simulink model "tdk_sim"  (R2017a)
settings: Solver=ode4  StartTime=0.0  StopTime=10  FixedStep=0.01  MaxStep=0.05  RelTol=1e-3  EnableMultiTasking=on
values from neighbouring files (symbols this model uses):
  x0_tdk = [0.5 0.5 0 0.1 0 0 0 0 0 0]    [tdk_sim_ini.m]
settings Model: Creator=ut  LastModifiedBy=maam
settings DataIOCC: LimitDataPoints=on  SaveFormat=Array  SignalLoggingSaveFormat=ModelDataLogs
settings OptimizationCC: ExpressionDepthLimit=2147483647  InitFltsAndDblsToZero=on  LifeSpan=inf
settings DebuggingCC: SaveWithParameterizedLinksMsg=none  UnderspecifiedInitializationDetection=Classic  MergeDetectMultiDrivingBlocksExec=none  SignalResolutionControl=TryResolveAllWithWarning  SolverPrmCheckMsg=warning  MultiTaskDSMMsg=warning  MultiTaskCondExecSysMsg=none  FcnCallInpInsideContextMsg=warning  StateNameClashWarn=warning  SFUnexpectedBacktrackingDiag=warning  SFNoUnconditionalDefaultTransitionDiag=warning  SFExecutionAtInitializationDiag=none
settings HardwareCC: ProdBitPerPointer=32  ProdBitPerSizeT=32  ProdBitPerPtrDiffT=32  ProdLargestAtomicFloat=None  ProdIntDivRoundTo=Undefined  ProdEndianess=Unspecified  ProdWordSize=32  ProdHWDeviceType=32-bit Generic
settings ModelReferenceCC: PropagateSignalLabelsOutOfModel=off
settings GRTTargetCC: TargetFcnLib=ansi_tfl_tmw.mat  TargetLangStandard=C89/C90 (ANSI)  CombineOutputUpdateFcns=off  GRTInterface=on
settings ConfigComp: CovMetricSettings=dw  CovSaveCumulativeToWorkspaceVar=on  CovSaveSingleToWorkspaceVar=on  CovExternalEMLEnable=off

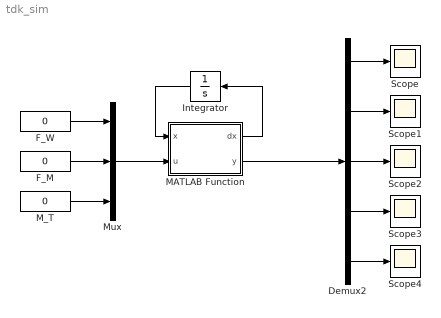
== system tdk_sim ==
  Demux2 : Demux  Outputs=5
  F_M : Constant  Value=0
  F_W : Constant  Value=0
  Integrator : Integrator  InitialCondition=x0_tdk
  MATLAB Function : MATLAB Function  TreatAsAtomicUnit=on
  M_T : Constant  Value=0
  Mux : Mux  Inputs=3
  Scope{,1..4} (5 alike) : Scope
  wires:
  MATLAB Function/2(y) -> Demux2/1
  Demux2/1 -> Scope/1
  Demux2/2 -> Scope1/1
  Demux2/3 -> Scope2/1
  Demux2/4 -> Scope3/1
  Demux2/5 -> Scope4/1
  MATLAB Function/1(dx) -> Integrator/1
  Integrator/1 -> MATLAB Function/1(x)
  F_W/1 -> Mux/1
  F_M/1 -> Mux/2
  M_T/1 -> Mux/3
  Mux/1 -> MATLAB Function/2(u)

== matlab function tdk_sim/MATLAB Function ==
  data: dx output; x input; y output; u input; par_tdk parameter
function [dx, y] = tdk_fcn(x, u, par_tdk)
%
% inputs:   u1(1)... F_W   Force of the cart [N]
%           u2(1)... F_M   Force of the rope winch [N]
%           u3(1)... M_T   Torque of the tower [Nm]
%
% states:   x(1)... l_W          Position of the cart [m]
%           x(2)... l_s          Rope length [m]
%           x(3)... phi_zi       Angle of the tower [rad]
%           x(4)... phi_xt       Angle of the load (x-axis) [rad]
%           x(5)... phi_yt       Angle of the load (y-axis) [rad]
%           x(6)... dot(l_W)     Velocity of the cart [m/s]
%           x(7)... dot(l_s)     Velocity of the rope [m/s]
%           x(8)... dot(phi_zi)  Angular velocity of the tower [rad/s]
%           x(9)... dot(phi_xt)  Angular velocity of the load (x-axis) [rad/s]
%           x(10)... dot(phi_yt) Angular velocity of the load (y-axis) [rad/s]
%
% outputs:  y(1)... l_W          Position of the cart [m]
%           y(2)... l_s          Rope length [m]
%           y(3)... phi_zi       Angle of the tower [rad]
%           y(4)... phi_xt       Angle of the load (x-axis) [rad]
%           y(5)... phi_yt       Angle of the load (y-axis) [rad]
%
% parameter: par_tdk(1)... m_M     Mass o the load m [kg]
%            par_tdk(2)... m_W     Mass of the cart
%            par_tdk(3)... m_TA    Mass of the tower-cantilever unit (TC-unit)
%            par_tdk(4)... k_M     Friction coefficient of the load
%            par_tdk(5)... k_TA    Friction coefficient of the load TC-unit
%            par_tdk(6)... k_W     Friction coefficient of the cart
%            par_tdk(7)... hTA     Height of the center of gravity of the TC-unit
%            par_tdk(8)... lTA     Distance of the center of gravity of the TC-unit in yi-direction
%            par_tdk(9)... J_Wzz   Inertia tensor of the cart
%            par_tdk(10)... J_TAzz Inertia tensor of the TC-unit
%            par_tdk(11)... g      Gravity acceleration
%    
    % Reading the model parameters               
    m_M = par_tdk(1); 
    m_W = par_tdk(2);  
    m_TA = par_tdk(3);  
    k_M = par_tdk(4); 
    k_TA = par_tdk(5); 
    k_W = par_tdk(6); 
    hTA = par_tdk(7); 
    lTA = par_tdk(8); 
    J_Wzz = par_tdk(9); 
    J_TAzz = par_tdk(10); 
    g = par_tdk(11);          

    % Shortcut for the inputs
    F_W = u(1);
    F_M = u(2);
    M_T = u(3);


    % Substitutions
    x_1 = x(1);
    x_2 = x(2);
    x_3 = x(3);
    x_4 = x(4);
    x_5 = x(5);
    x_6 = x(6);
    x_7 = x(7);
    x_8 = x(8);
    x_9 = x(9);
    x_10 = x(10);  

    % Calculation of the states time derivative
    dx = zeros(10, 1);
    dx(1) = x_6;
    dx(2) = x_7;
    dx(3) = x_8;
    dx(4) = x_9;
    dx(5) = x_10;
    dx(6) = (x_1*x_2*x_8^2*m_W-x_2*x_6*k_W-cos(x_4)*x_9*k_M+x_2*F_W)/(x_2*m_W);
    dx(7) = (x_1*x_2*cos(x_4)*sin(x_5)*m_M*m_W*M_T+(x_1^2*(x_2^2*(x_9^2+x_8*(2*sin(x_5)*x_9-2*x_10*cos(x_4)*sin(x_4)*cos(x_5))+(1-cos(x_4)^2*cos(x_5)^2)*x_8^2+x_10^2*cos(x_4)^2)+g*x_2*cos(x_4)*cos(x_5))*m_M-x_1^2*x_2*F_M)*m_W^2+((((x_2^2*(x_9^2+x_8*(2*sin(x_5)*x_9-2*x_10*cos(x_4)*sin(x_4)*cos(x_5))+(1-cos(x_4)^2*cos(x_5)^2)*x_8^2+x_10^2*cos(x_4)^2)+g*x_2*cos(x_4)*cos(x_5))*lTA^2-2*x_2*cos(x_4)*sin(x_5)*x_6*x_8*lTA^2)*m_M-x_2*F_M*lTA^2)*m_TA+(x_6*((-2*J_Wzz-2*J_TAzz)*x_2*cos(x_4)*sin(x_5)*x_8-x_1^2*x_2*sin(x_4)*k_W)+x_1*x_2*(cos(x_4)*sin(x_5)*x_8*k_TA+(cos(x_4)*cos(x_5)^2*x_9-cos(x_4)*x_9+x_10*sin(x_4)*cos(x_5)*sin(x_5))*k_M)+x_1^2*((-cos(x_4)*sin(x_4)*cos(x_5)^2*x_9-x_10*cos(x_5)*sin(x_5))*k_M+x_2*sin(x_4)*F_W)+x_2^2*((J_Wzz+J_TAzz)*x_9^2+x_8*((2*J_Wzz+2*J_TAzz)*sin(x_5)*x_9+(-2*J_Wzz-2*J_TAzz)*x_10*cos(x_4)*sin(x_4)*cos(x_5))+((-J_Wzz-J_TAzz)*cos(x_4)^2*cos(x_5)^2+J_Wzz+J_TAzz)*x_8^2+(J_Wzz+J_TAzz)*x_10^2*cos(x_4)^2)+(g*J_Wzz+g*J_TAzz)*x_2*cos(x_4)*cos(x_5))*m_M+(-J_Wzz-J_TAzz)*x_2*F_M)*m_W+((x_2*sin(x_4)*F_W-cos(x_4)*sin(x_4)*x_9*k_M)*lTA^2-x_2*sin(x_4)*x_6*k_W*lTA^2)*m_M*m_TA+((-J_Wzz-J_TAzz)*x_2*sin(x_4)*x_6*k_W+(-J_Wzz-J_TAzz)*cos(x_4)*sin(x_4)*x_9*k_M+(J_Wzz+J_TAzz)*x_2*sin(x_4)*F_W)*m_M)/(x_1^2*x_2*m_M*m_W^2+(x_2*lTA^2*m_M*m_TA+(J_Wzz+J_TAzz)*x_2*m_M)*m_W);
    dx(8) = -(x_2*cos(x_4)*M_T+2*x_1*x_2*cos(x_4)*x_6*x_8*m_W+x_2*(cos(x_4)*x_8*k_TA+(x_10*sin(x_4)*cos(x_5)-cos(x_4)*sin(x_5)*x_9)*k_M)+x_1*(cos(x_4)*sin(x_4)*sin(x_5)*x_9-x_10*cos(x_5))*k_M)/(x_1^2*x_2*cos(x_4)*m_W+x_2*cos(x_4)*lTA^2*m_TA+(J_Wzz+J_TAzz)*x_2*cos(x_4));
    dx(9) = -((x_1*x_2*cos(x_4)*sin(x_4)*sin(x_5)-x_2^2*cos(x_4)*sin(x_5))*m_M*m_W*M_T+((x_1^2*(x_2*x_7*(2*cos(x_4)*x_9+2*cos(x_4)*sin(x_5)*x_8)+x_2^2*(-cos(x_4)^2*sin(x_4)*cos(x_5)^2*x_8^2+2*x_10*cos(x_4)^3*cos(x_5)*x_8+x_10^2*cos(x_4)^2*sin(x_4))+g*x_2*cos(x_4)*sin(x_4)*cos(x_5))-2*x_1*x_2^2*cos(x_4)*sin(x_5)*x_6*x_8)*m_M+x_1^2*cos(x_4)*x_9*k_M)*m_W^2+((((x_2*x_7*(2*cos(x_4)*x_9+2*cos(x_4)*sin(x_5)*x_8)+x_2^2*(-cos(x_4)^2*sin(x_4)*cos(x_5)^2*x_8^2+2*x_10*cos(x_4)^3*cos(x_5)*x_8+x_10^2*cos(x_4)^2*sin(x_4))+g*x_2*cos(x_4)*sin(x_4)*cos(x_5))*lTA^2-2*x_2*cos(x_4)*sin(x_4)*sin(x_5)*x_6*x_8*lTA^2)*m_M+cos(x_4)*x_9*k_M*lTA^2)*m_TA+(x_6*(x_1^2*x_2*cos(x_4)^2*k_W+(-2*J_Wzz-2*J_TAzz)*x_2*cos(x_4)*sin(x_4)*sin(x_5)*x_8)+x_1*x_2*(cos(x_4)*sin(x_4)*sin(x_5)*x_8*k_TA+(x_10*(sin(x_4)^2+1)*cos(x_5)*sin(x_5)-2*cos(x_4)*sin(x_4)*sin(x_5)^2*x_9)*k_M)+x_2^2*(-cos(x_4)*sin(x_5)*x_8*k_TA+(cos(x_4)*sin(x_5)^2*x_9-x_10*sin(x_4)*cos(x_5)*sin(x_5))*k_M+(-J_Wzz-J_TAzz)*cos(x_4)^2*sin(x_4)*cos(x_5)^2*x_8^2+(2*J_Wzz+2*J_TAzz)*x_10*cos(x_4)^3*cos(x_5)*x_8+(J_Wzz+J_TAzz)*x_10^2*cos(x_4)^2*sin(x_4))+x_1^2*((cos(x_4)*sin(x_4)^2*sin(x_5)^2*x_9+cos(x_4)^3*x_9-x_10*sin(x_4)*cos(x_5)*sin(x_5))*k_M-x_2*cos(x_4)^2*F_W)+x_2*x_7*((2*J_Wzz+2*J_TAzz)*cos(x_4)*x_9+(2*J_Wzz+2*J_TAzz)*cos(x_4)*sin(x_5)*x_8)+(g*J_Wzz+g*J_TAzz)*x_2*cos(x_4)*sin(x_4)*cos(x_5))*m_M+(J_Wzz+J_TAzz)*cos(x_4)*x_9*k_M)*m_W+(x_2*cos(x_4)^2*x_6*k_W*lTA^2+(cos(x_4)^3*x_9*k_M-x_2*cos(x_4)^2*F_W)*lTA^2)*m_M*m_TA+((J_Wzz+J_TAzz)*x_2*cos(x_4)^2*x_6*k_W+(J_Wzz+J_TAzz)*cos(x_4)^3*x_9*k_M+(-J_Wzz-J_TAzz)*x_2*cos(x_4)^2*F_W)*m_M)/(x_1^2*x_2^2*cos(x_4)*m_M*m_W^2+(x_2^2*cos(x_4)*lTA^2*m_M*m_TA+(J_Wzz+J_TAzz)*x_2^2*cos(x_4)*m_M)*m_W);
    dx(10) = ((x_1*x_2*cos(x_4)*cos(x_5)-x_2^2*cos(x_4)*sin(x_4)*cos(x_5))*m_M*M_T+((x_1^2*(x_2^2*(2*cos(x_4)^2*cos(x_5)*x_8*x_9+2*x_10*cos(x_4)*sin(x_4)*x_9+cos(x_4)^2*cos(x_5)*sin(x_5)*x_8^2)+x_2*x_7*(2*cos(x_4)*sin(x_4)*cos(x_5)*x_8-2*x_10*cos(x_4)^2)-g*x_2*cos(x_4)*sin(x_5))-2*x_1*x_2^2*cos(x_4)*sin(x_4)*cos(x_5)*x_6*x_8)*m_M-x_1^2*x_10*k_M)*m_W+(((x_2^2*(2*cos(x_4)^2*cos(x_5)*x_8*x_9+2*x_10*cos(x_4)*sin(x_4)*x_9+cos(x_4)^2*cos(x_5)*sin(x_5)*x_8^2)+x_2*x_7*(2*cos(x_4)*sin(x_4)*cos(x_5)*x_8-2*x_10*cos(x_4)^2)-g*x_2*cos(x_4)*sin(x_5))*lTA^2-2*x_2*cos(x_4)*cos(x_5)*x_6*x_8*lTA^2)*m_M-x_10*k_M*lTA^2)*m_TA+(x_2^2*(-cos(x_4)*sin(x_4)*cos(x_5)*x_8*k_TA+(cos(x_4)*sin(x_4)*cos(x_5)*sin(x_5)*x_9+x_10*(cos(x_4)^2-1)*cos(x_5)^2)*k_M+(2*J_Wzz+2*J_TAzz)*cos(x_4)^2*cos(x_5)*x_8*x_9+(2*J_Wzz+2*J_TAzz)*x_10*cos(x_4)*sin(x_4)*x_9+(J_Wzz+J_TAzz)*cos(x_4)^2*cos(x_5)*sin(x_5)*x_8^2)+x_1*x_2*(cos(x_4)*cos(x_5)*x_8*k_TA+((cos(x_4)^3-2*cos(x_4))*cos(x_5)*sin(x_5)*x_9+2*x_10*sin(x_4)*cos(x_5)^2)*k_M)+x_1^2*(cos(x_4)*sin(x_4)*cos(x_5)*sin(x_5)*x_9-x_10*cos(x_5)^2)*k_M+x_2*x_7*((2*J_Wzz+2*J_TAzz)*cos(x_4)*sin(x_4)*cos(x_5)*x_8+(-2*J_Wzz-2*J_TAzz)*x_10*cos(x_4)^2)+(-2*J_Wzz-2*J_TAzz)*x_2*cos(x_4)*cos(x_5)*x_6*x_8+(-g*J_Wzz-g*J_TAzz)*x_2*cos(x_4)*sin(x_5))*m_M+(-J_Wzz-J_TAzz)*x_10*k_M)/(x_1^2*x_2^2*cos(x_4)^2*m_M*m_W+x_2^2*cos(x_4)^2*lTA^2*m_M*m_TA+(J_Wzz+J_TAzz)*x_2^2*cos(x_4)^2*m_M);

    % Assingment of the outputs
    y = zeros(5, 1);
    y(1) = x(1);
    y(2) = x(2);
    y(3) = x(3); 
    y(4) = x(4);
    y(5) = x(5);
